simulink model "sim_battery_system"  (R2018b)
settings: Solver=FixedStepDiscrete  StartTime=0.0  StopTime=SimPara.t_sim  FixedStep=SimPara.t_step  RelTol=1e-3
undefined symbols (not defined in the file or in its folder): A, BatPara, i, LSAPara, p, SimPara, SysPara, x2_cal, x3_cal, x_cal
libraries: simulink x14, dspstat3 x4, dspindex x1
(part 4 of 4)

== system sim_battery_system/Monitoring and Logging/Load Spectrum Analysis/Load Spectrum Analysis ON/Load Spectrum Analysis ON/Two parametric LSA of cell SOC vs. temperature /For Iterator val1/For Iterator val2  ==
  rfk1 : Inport
  val2_in : Inport  Port=2
  k : Inport  Port=3
  data_in_delayed : Inport  Port=4
  bins_val2 : Inport  Port=5
  Add1 : Sum
  Assignment Subsystem : Subsystem  TreatAsAtomicUnit=on
  Constant1 : Constant  Value=bins_borders_2
  Constant4 : Constant
  Find Nonzero Elements : Find
  Iterate number of bins val2 : ForIterator  ResetStates=reset  IterationSource=external  IterationLimit=length(x_cal)  IterationVariableDataType=double
  Logical Operator : Logic  AllPortsSameDT=off  OutDataTypeStr=boolean
  Relational Operator : RelationalOperator  OutDataTypeStr=boolean  RndMeth=Simplest
  Relational Operator1 : RelationalOperator  Operator=<  OutDataTypeStr=boolean  RndMeth=Simplest
  Reshape : Reshape
  Selector : Selector  InputPortWidth=SysPara.p*SysPara.s  IndexOptions=Index vector (port)  Indices=[1 3]  OutputSizes=1
  select cells in the SOC- Range corresponding to 1. FOR Iterator : Selector  InputPortWidth=SysPara.p*SysPara.s  IndexOptions=Index vector (port)  Indices=1:p  OutputSizes=1
  select parallel cell1 : Selector  InputPortWidth=length(bins_borders_2)  IndexOptions=Index vector (port)  Indices=1:p  OutputSizes=1
  select parallel cell2 : Selector  InputPortWidth=length(bins_borders_2)  IndexOptions=Index vector (port)  Indices=1:p  OutputSizes=1
  LSA_out : Outport
  wires:
  bins_val2/1 -> Iterate number of bins val2/1
  data_in_delayed/1 -> Assignment Subsystem/4(data_in_delayed)
  Constant1/1 -> select parallel cell1/1, select parallel cell2/1
  Iterate number of bins val2/1 -> select parallel cell2/2, Assignment Subsystem/2(a), Add1/2
  Add1/1 -> select parallel cell1/2
  Constant4/1 -> Add1/1
  select parallel cell2/1 -> Relational Operator/2
  select parallel cell1/1 -> Relational Operator1/2
  Relational Operator1/1 -> Logical Operator/2
  Relational Operator/1 -> Logical Operator/1
  select cells in the SOC- Range corresponding to 1. FOR Iterator/1 -> Relational Operator1/1, Relational Operator/1
  k/1 -> Assignment Subsystem/1(k)
  val2_in/1 -> Reshape/1
  Reshape/1 -> select cells in the SOC- Range corresponding to 1. FOR Iterator/1
  Logical Operator/1 -> Find Nonzero Elements/1
  rfk1/1 -> Selector/1, select cells in the SOC- Range corresponding to 1. FOR Iterator/2
  Find Nonzero Elements/1 -> Selector/2
  Selector/1 -> Assignment Subsystem/3(index_cell)
  Assignment Subsystem/1(LSA_out) -> LSA_out/1

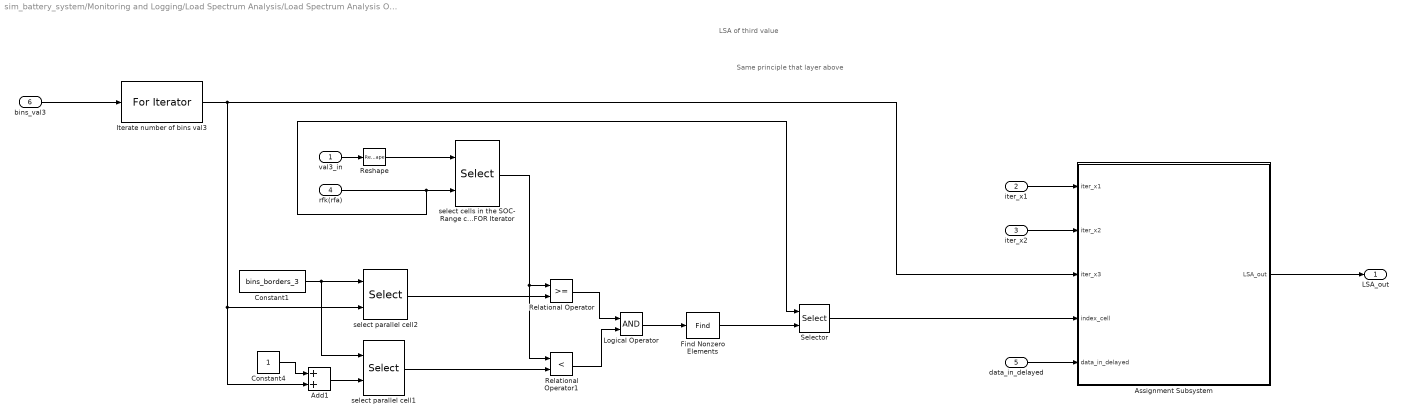
== system sim_battery_system/Monitoring and Logging/Load Spectrum Analysis/Load Spectrum Analysis ON/Load Spectrum Analysis ON/3-parametrische Momentanwertzählung SOC, T_Cells, CRate/For Iterator val1/For Iterator val2/For Iterator CRate ==
  note: Same principle that layer above
  note: LSA of third value
  val3_in : Inport
  iter_x1 : Inport  Port=2
  iter_x2 : Inport  Port=3
  rfk(rfa) : Inport  Port=4
  data_in_delayed : Inport  Port=5
  bins_val3 : Inport  Port=6
  Add1 : Sum
  Assignment Subsystem : Subsystem  TreatAsAtomicUnit=on
  Constant1 : Constant  Value=bins_borders_3
  Constant4 : Constant
  Find Nonzero Elements : Find
  Iterate number of bins val3 : ForIterator  ResetStates=reset  IterationSource=external  IterationLimit=length(x3_cal)  IterationVariableDataType=double
  Logical Operator : Logic  AllPortsSameDT=off  OutDataTypeStr=boolean
  Relational Operator : RelationalOperator  OutDataTypeStr=boolean  RndMeth=Simplest
  Relational Operator1 : RelationalOperator  Operator=<  OutDataTypeStr=boolean  RndMeth=Simplest
  Reshape : Reshape
  Selector : Selector  InputPortWidth=SysPara.p*SysPara.s  IndexOptions=Index vector (port)  Indices=[1 3]  OutputSizes=1
  select cells in the SOC- Range corresponding to 1. FOR Iterator : Selector  InputPortWidth=SysPara.p*SysPara.s  IndexOptions=Index vector (port)  Indices=1:p  OutputSizes=1
  select parallel cell1 : Selector  InputPortWidth=length(bins_borders_3)  IndexOptions=Index vector (port)  Indices=1:p  OutputSizes=1
  select parallel cell2 : Selector  InputPortWidth=length(bins_borders_3)  IndexOptions=Index vector (port)  Indices=1:p  OutputSizes=1
  LSA_out : Outport
  wires:
  Find Nonzero Elements/1 -> Selector/2
  bins_val3/1 -> Iterate number of bins val3/1
  rfk(rfa)/1 -> select cells in the SOC- Range corresponding to 1. FOR Iterator/2, Selector/1
  Logical Operator/1 -> Find Nonzero Elements/1
  Reshape/1 -> select cells in the SOC- Range corresponding to 1. FOR Iterator/1
  val3_in/1 -> Reshape/1
  select cells in the SOC- Range corresponding to 1. FOR Iterator/1 -> Relational Operator/1, Relational Operator1/1
  Relational Operator/1 -> Logical Operator/1
  Relational Operator1/1 -> Logical Operator/2
  select parallel cell1/1 -> Relational Operator1/2
  select parallel cell2/1 -> Relational Operator/2
  Constant4/1 -> Add1/1
  Add1/1 -> select parallel cell1/2
  Iterate number of bins val3/1 -> select parallel cell2/2, Add1/2, Assignment Subsystem/3(iter_x3)
  Constant1/1 -> select parallel cell2/1, select parallel cell1/1
  iter_x2/1 -> Assignment Subsystem/2(iter_x2)
  Assignment Subsystem/1(LSA_out) -> LSA_out/1
  iter_x1/1 -> Assignment Subsystem/1(iter_x1)
  data_in_delayed/1 -> Assignment Subsystem/5(data_in_delayed)
  Selector/1 -> Assignment Subsystem/4(index_cell)

== system sim_battery_system/Monitoring and Logging/Load Spectrum Analysis/Load Spectrum Analysis ON/Load Spectrum Analysis ON/Two parametric LSA of cell C-Rate vs. temperature/For Iterator val1/For Iterator val2 /Assignment Subsystem ==
  k : Inport
  a : Inport  Port=2
  index_cell : Inport  Port=3
  data_in_delayed : Inport  Port=4
  Add : Sum
  Assignment of matrix entries : Assignment  NumberOfDimensions=3  OutputInitialize=Specify size for each dimension in table  IndexOptions=Index vector (port),Index vector (port),Index vector (port)  Indices=1,1,1  OutputSizes=length(bins_mean_1),length(bins_mean_2),SysPara.p*SysPara.s+1
  Constant1 : Constant  Value=SimPara.t_step
  "Selection of delayed matrix entries " : Selector  NumberOfDimensions=3  InputPortWidth=3  IndexOptions=Index vector (port),Index vector (port),Index vector (port)  Indices=[1 3],1,1  OutputSizes=1,1,1
  LSA_out : Outport
  wires:
  index_cell/1 -> "Selection of delayed matrix entries "/4, Assignment of matrix entries/4
  Assignment of matrix entries/1 -> LSA_out/1
  a/1 -> Assignment of matrix entries/3, "Selection of delayed matrix entries "/3
  k/1 -> Assignment of matrix entries/2, "Selection of delayed matrix entries "/2
  Constant1/1 -> Add/1
  "Selection of delayed matrix entries "/1 -> Add/2
  Add/1 -> Assignment of matrix entries/1
  data_in_delayed/1 -> "Selection of delayed matrix entries "/1

== system sim_battery_system/Monitoring and Logging/Load Spectrum Analysis/Load Spectrum Analysis ON/Load Spectrum Analysis ON/Two parametric LSA of cell SOC vs. C-Rate/For Iterator val1/For Iterator val2 /Assignment Subsystem ==
  k : Inport
  a : Inport  Port=2
  index_cell : Inport  Port=3
  data_in_delayed : Inport  Port=4
  Add : Sum
  Assignment of matrix entries : Assignment  NumberOfDimensions=3  OutputInitialize=Specify size for each dimension in table  IndexOptions=Index vector (port),Index vector (port),Index vector (port)  Indices=1,1,1  OutputSizes=length(bins_mean_1),length(bins_mean_2),SysPara.p*SysPara.s+1
  Constant1 : Constant  Value=SimPara.t_step
  "Selection of delayed matrix entries " : Selector  NumberOfDimensions=3  InputPortWidth=3  IndexOptions=Index vector (port),Index vector (port),Index vector (port)  Indices=[1 3],1,1  OutputSizes=1,1,1
  LSA_out : Outport
  wires:
  data_in_delayed/1 -> "Selection of delayed matrix entries "/1
  Add/1 -> Assignment of matrix entries/1
  "Selection of delayed matrix entries "/1 -> Add/2
  Constant1/1 -> Add/1
  k/1 -> "Selection of delayed matrix entries "/2, Assignment of matrix entries/2
  a/1 -> "Selection of delayed matrix entries "/3, Assignment of matrix entries/3
  Assignment of matrix entries/1 -> LSA_out/1
  index_cell/1 -> Assignment of matrix entries/4, "Selection of delayed matrix entries "/4

== system sim_battery_system/Monitoring and Logging/Load Spectrum Analysis/Load Spectrum Analysis ON/Load Spectrum Analysis ON/Two parametric LSA of cell SOC vs. temperature /For Iterator val1/For Iterator val2 /Assignment Subsystem ==
  k : Inport
  a : Inport  Port=2
  index_cell : Inport  Port=3
  data_in_delayed : Inport  Port=4
  Add : Sum
  Assignment of matrix entries : Assignment  NumberOfDimensions=3  OutputInitialize=Specify size for each dimension in table  IndexOptions=Index vector (port),Index vector (port),Index vector (port)  Indices=1,1,1  OutputSizes=length(bins_mean_1),length(bins_mean_2),SysPara.p*SysPara.s+1
  Constant1 : Constant  Value=SimPara.t_step
  "Selection of delayed matrix entries " : Selector  NumberOfDimensions=3  InputPortWidth=3  IndexOptions=Index vector (port),Index vector (port),Index vector (port)  Indices=[1 3],1,1  OutputSizes=1,1,1
  LSA_out : Outport
  wires:
  data_in_delayed/1 -> "Selection of delayed matrix entries "/1
  Add/1 -> Assignment of matrix entries/1
  "Selection of delayed matrix entries "/1 -> Add/2
  Constant1/1 -> Add/1
  k/1 -> "Selection of delayed matrix entries "/2, Assignment of matrix entries/2
  a/1 -> "Selection of delayed matrix entries "/3, Assignment of matrix entries/3
  Assignment of matrix entries/1 -> LSA_out/1
  index_cell/1 -> Assignment of matrix entries/4, "Selection of delayed matrix entries "/4

== system sim_battery_system/Monitoring and Logging/Load Spectrum Analysis/Load Spectrum Analysis ON/Load Spectrum Analysis ON/3-parametrische Momentanwertzählung SOC, T_Cells, CRate/For Iterator val1/For Iterator val2/For Iterator CRate/Assignment Subsystem ==
  note: Assign updated value to tensor of last time-step
  note: Select field that will get updated in this time-step
  iter_x1 : Inport
  iter_x2 : Inport  Port=2
  iter_x3 : Inport  Port=3
  index_cell : Inport  Port=4
  data_in_delayed : Inport  Port=5
  Add : Sum
  Assignment of matrix entries : Assignment  NumberOfDimensions=4  OutputInitialize=Specify size for each dimension in table  IndexOptions=Index vector (port),Index vector (port),Index vector (port),Index vector (port)  Indices=1,1,1,1  OutputSizes=length(bins_mean_1),length(bins_mean_2),length(bins_mean_3),SysPara.p*SysPara.s+1
  Constant1 : Constant  Value=SimPara.t_step
  "Selection of delayed matrix entries " : Selector  NumberOfDimensions=4  InputPortWidth=3  IndexOptions=Index vector (port),Index vector (port),Index vector (port),Index vector (port)  Indices=[1 3],1,1,1  OutputSizes=1,1,1,1
  LSA_out : Outport
  wires:
  iter_x3/1 -> Assignment of matrix entries/4, "Selection of delayed matrix entries "/4
  index_cell/1 -> "Selection of delayed matrix entries "/5, Assignment of matrix entries/5
  Assignment of matrix entries/1 -> LSA_out/1
  iter_x2/1 -> Assignment of matrix entries/3, "Selection of delayed matrix entries "/3
  iter_x1/1 -> Assignment of matrix entries/2, "Selection of delayed matrix entries "/2
  Constant1/1 -> Add/1
  "Selection of delayed matrix entries "/1 -> Add/2
  Add/1 -> Assignment of matrix entries/1
  data_in_delayed/1 -> "Selection of delayed matrix entries "/1
